simulink model "S2DOFSP"  (R2023a)
settings: Solver=VariableStepAuto  StartTime=0.0  StopTime=Tsim  RelTol=1e-3
values from neighbouring files (symbols this model uses):
  s = tf('s')    [DTCoBSERVER.m]
undefined symbols (not defined in the file or in its folder): Ampdist, Gn, L, Tdist, Tinit
libraries: cstblocks x7, simulink x1
settings Model: Creator=jprmj  LastModifiedBy=juan
settings OptimizationCC: ReuseModelBlockBuffer=off

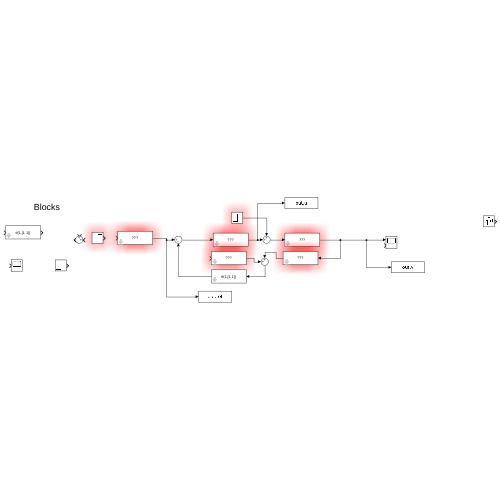
[thumbnail: Simulink's stored preview of the top-level diagram]
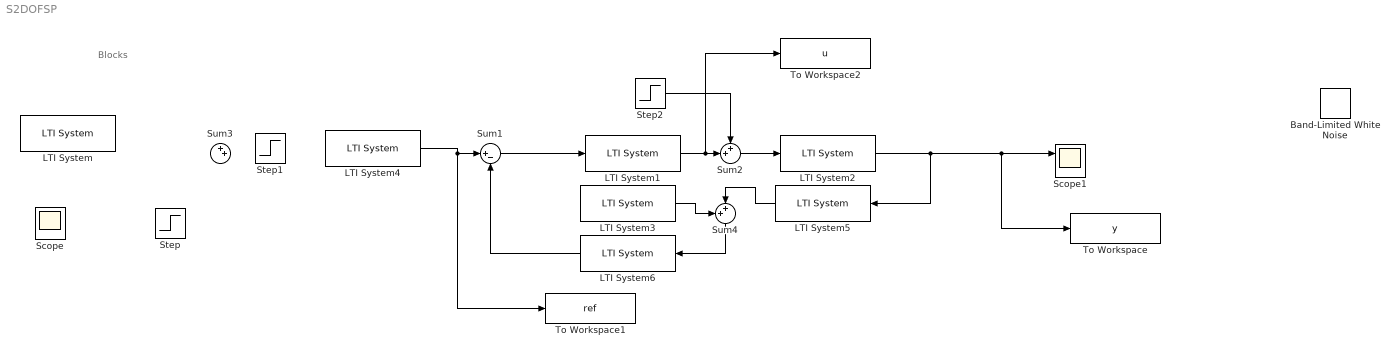
== system S2DOFSP ==
  note: Blocks
  Band-Limited White Noise : simulink/Sources/Band-Limited White Noise  Cov=[0.1]  Ts=0.1  seed=[23341]
  LTI System : cstblocks/LTI System  sys=tf(1,[1 1])  IC=[]
  LTI System1 : cstblocks/LTI System  sys=C_sp  IC=[]
  LTI System2 : cstblocks/LTI System  sys=P  IC=[]
  LTI System3 : cstblocks/LTI System  sys=exp(-L*s)  IC=[]
  LTI System4 : cstblocks/LTI System  sys=F  IC=[]
  LTI System5 : cstblocks/LTI System  sys=Gn-1  IC=[]
  LTI System6 : cstblocks/LTI System  sys=tf(1,[1 1])  IC=[]
  Scope : Scope
  Scope1 : Scope  NumInputPorts=2
  Step : Step  SampleTime=0
  Step1 : Step  SampleTime=Tinit
  Step2 : Step  After=Ampdist  SampleTime=Tdist
  Sum1 : Sum  Inputs=|+-
  Sum2 : Sum  Inputs=++|
  Sum3 : Sum  Inputs=++|
  Sum4 : Sum  Inputs=++|
  To Workspace : ToWorkspace  VariableName=y  SaveFormat=Timeseries  SampleTime=-1
  To Workspace1 : ToWorkspace  VariableName=ref  SaveFormat=Timeseries  SampleTime=-1
  To Workspace2 : ToWorkspace  VariableName=u  SaveFormat=Timeseries  SampleTime=-1
  wires:
  Sum2/1 -> LTI System2/1
  LTI System1/1 -> To Workspace2/1, Sum2/2
  LTI System2/1 -> LTI System5/1, To Workspace/1, Scope1/1
  Step2/1 -> Sum2/1
  LTI System4/1 -> To Workspace1/1, Sum1/1
  Sum1/1 -> LTI System1/1
  LTI System3/1 -> Sum4/1
  LTI System5/1 -> Sum4/2
  Sum4/1 -> LTI System6/1
  LTI System6/1 -> Sum1/2
